simulink model "ex7busLongLine_sim"  (R2014b)
settings: Solver=ode45  SolverMode=SingleTasking  StartTime=0.0  StopTime=5  MaxStep=0.0005  RelTol=1e-07
values from neighbouring files (symbols this model uses):
  bus1_vd = 2^0.5*1e3    (= 1414.21356237)    [ex3busPV.m]    (also in exLongLinePV.m = 141421.356237)
  C2 = 0.1*(len12/NN12+len23/NN23+len25/NN25)*Cx    (= 7.75146666667e-08)    [ex7busLongLine.m]
  C3 = 0.1*(len23/NN23+len34/NN34)*Cx    (= 3.50675e-08)    [ex7busLongLine.m]
  C4 = 0.1*(len14/NN14+len34/NN34+len46/NN46)*Cx    (= 9.28655e-08)    [ex7busLongLine.m]
  C5 = 0.1*(len25/NN25)*Cx    (= 2.39416666667e-08)    [ex7busLongLine.m]
  C6 = 0.1*(len46/NN46+len67/NN67)*Cx    (= 4.85875e-08)    [ex7busLongLine.m]
  C7 = 0.1*(len67/NN67)*Cx    (= 2.66175e-08)    [ex7busLongLine.m]
  CL2 = -CL2    [ex7busLongLine.m]
  CL3 = -CL3    [ex7busLongLine.m]
  CL6 = -CL6    [ex7busLongLine.m]
  CL7 = -CL7    [ex7busLongLine.m]
  DL2 = -DL2    [ex7busLongLine.m]
  DL3 = -DL3    [ex7busLongLine.m]
  DL6 = -DL6    [ex7busLongLine.m]
  DL7 = -DL7    [ex7busLongLine.m]
  droop_Pref = 0.25*Pbase    (= 75000000)    [ex7busLongLine.m]    (also in exDroopA.m = mpc.gen(2:end,PG)*1e6; exDroopB.m = mpc.gen(:,PG)*1e6; exSyncGenPVinv.m = droop_Pref( [1:(synrp-1),(synrp+1):end]  ))
  droop_R = DROOP_R_GAIN_CNST./Prt    [ex7busLongLine.m]    (also in exDroopA.m; exDroopB.m)
  Epv = 22e3    (= 22000)    [ex7busLongLine.m]
  If_dc = 0.2*Prt./Ert    [ex14busSGandPV.m]    (also in ex7busLongLine.m = Prt./(60*Vf_dc); exDroopA.m = Prt./(60*Vf_dc); exDroopB.m = Prt./(60*Vf_dc); exSyncGenPVinv.m)
  Jpv = JPV_CNST*Ppvrt/ws    (= 95.4929658551)    [ex7busLongLine.m]
  Kd = KD_GAIN_CNST*J*ws    [ex14busSGandPV.m]    (also in ex2busStability.m = 24000; ex7busLongLine.m; ex9busSG.m; exDroopA.m)
  Kdpv = KDPV_CNST*Jpv*ws    (= 6000000)    [ex7busLongLine.m]
  L0 = 0.1*Ld    [ex14busSGandPV.m]    (also in ex7busLongLine.m; exDroopA.m; exDroopB.m; exSyncGenPVinv.m)
  Laf = (2^0.5)*Ert./(ws*If_dc)    [ex14busSGandPV.m]    (also in ex7busLongLine.m; exDroopA.m; exDroopB.m; exSyncGenPVinv.m = (2^0.5)*5*Ert.^2./(ws*Prt))
  Lb2 = 2*Ld.*Lff - 3*Laf.^2    [ex14busSGandPV.m]    (also in ex7busLongLine.m; exDroopA.m; exDroopB.m; exSyncGenPVinv.m)
  Ld = 0.6*Lpu    [ex14busSGandPV.m]    (also in ex7busLongLine.m = 0.3*Lpu; exDroopA.m = 0.3*Lpu; exDroopB.m = 0.3*Lpu; exSyncGenPVinv.m)
  Lff = 2*Laf.^2./Ld    [ex14busSGandPV.m]    (also in ex7busLongLine.m; exDroopA.m; exDroopB.m; exSyncGenPVinv.m)
  Lq = Ld    [ex14busSGandPV.m]    (also in ex7busLongLine.m; exDroopA.m; exDroopB.m; exSyncGenPVinv.m)
  Lspv = 0.1*Epv^2/(Ppvrt*ws)    (= 0.00256769974855)    [ex7busLongLine.m]
  PG5 = 0.8*Ppvrt    (= 48000000)    [ex7busLongLine.m]
  poles_2Jws = poles./(2*J*ws)    [ex14busSGandPV.m]    (also in ex2busStability.m = poles./(2*ws*J); ex7busLongLine.m; ex9busSG.m = poles./(2*ws*J); exDroopA.m)
  Ra = 0.05*Ert.^2./Prt    [ex14busSGandPV.m]    (also in ex7busLongLine.m = 0.01*Ert.^2./Prt; exDroopA.m = 0.01*Ert.^2./Prt; exDroopB.m = 0.01*Ert.^2./Prt; exSyncGenPVinv.m)
  rel_step_4 = 0.5    [ex7busLongLine.m]
  rel_step_5 = -0.5    [ex7busLongLine.m]
  Rf = Lff/1.2    [ex14busSGandPV.m]    (also in ex7busLongLine.m = Vf_dc./If_dc; exDroopA.m = Vf_dc./If_dc; exDroopB.m = Vf_dc./If_dc; exSyncGenPVinv.m)
  tratio4 = 22e3 / Vbase    (= 0.136645962733)    [ex7busLongLine.m]
  tratio5 = 22e3 / Vbase    (= 0.136645962733)    [ex7busLongLine.m]
  tss2 = 4.5    [ex7busLongLine.m]
  tss3 = 1e9    (= 1000000000)    [ex7busLongLine.m]
  tss4 = 1e9    (= 1000000000)    [ex7busLongLine.m]
  tss5 = 4    [ex7busLongLine.m]
  tss6 = 1e9    (= 1000000000)    [ex7busLongLine.m]
  tss7 = 1e9    (= 1000000000)    [ex7busLongLine.m]
  Vbase = 161e3    (= 161000)    [ex7busLongLine.m]
  Vf_dc = If_dc.*Rf    [ex14busSGandPV.m]    (also in ex7busLongLine.m = 500 * ones(size(Ert)); exDroopA.m = 500 * ones(size(Ert)); exDroopB.m = 500 * ones(size(Ert)); exSyncGenPVinv.m)
  vinf_0 = 0    [ex14busSGandPV.m]    (also in ex7busLongLine.m; exDroopA.m; exSyncGenPVinv.m)
  vinf_d = (2^0.5)*mpcA.bus(1,VM)*baseV    [ex14busSGandPV.m]    (also in ex7busLongLine.m = 250457.221896; exDroopA.m = (2^0.5)*mpc.bus(1,VM)*baseV(1); exSyncGenPVinv.m = (2^0.5)*mpc.bus(1,VM)*baseV(1))
  vinf_q = 0    [ex14busSGandPV.m]    (also in ex7busLongLine.m; exDroopA.m; exSyncGenPVinv.m)
  ws = 2*pi*50    (= 314.159265359)    [ex14busSGandPV.m]    (also in ex2busStability.m; ex3busPV.m; ex7busLongLine.m; ex9busSG.m)
undefined symbols (not defined in the file or in its folder): AL2, AL3, AL6, AL7, At12, At14, At23, At25, At34, At46, At67, BL2, BL3, BL6, BL7, Bt12, Bt14, Bt23, Bt25, Bt34, Bt46, Bt67, Ct12, Ct14, Ct23, Ct25, Ct34, Ct46, Ct67, Dt12, Dt14, Dt23, Dt25, Dt34, Dt46, Dt67, full
(part 1 of 2)
settings Model: Creator=COPEC  LastModifiedBy=Juri
settings OptimizationCC: BlockReduction=off  BooleanDataType=off
settings DebuggingCC: SaveWithParameterizedLinksMsg=none  UnderspecifiedInitializationDetection=Classic  MergeDetectMultiDrivingBlocksExec=none  SignalResolutionControl=TryResolveAllWithWarning  SolverPrmCheckMsg=none  FrameProcessingCompatibilityMsg=error
settings HardwareCC: TargetUnknown=on

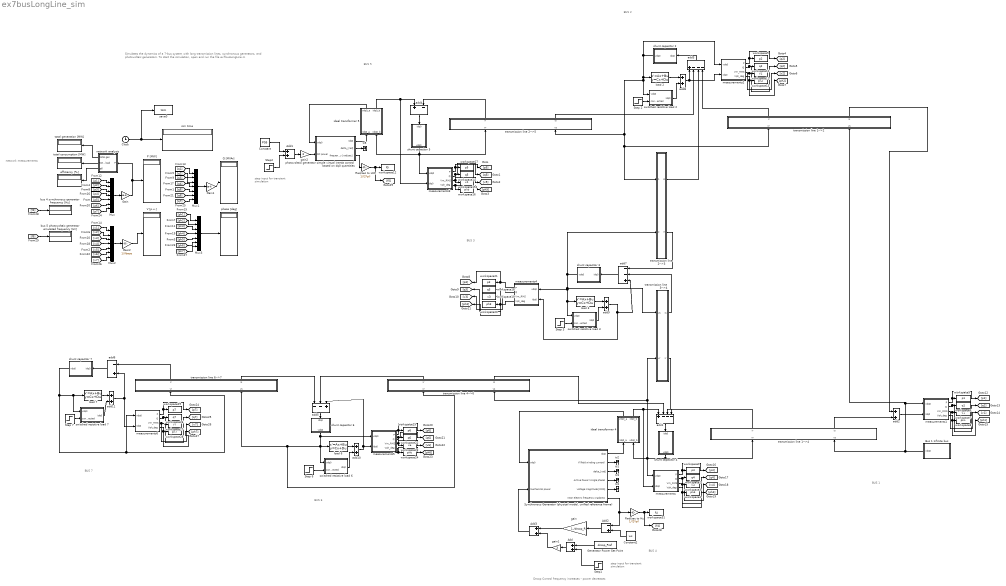
== system ex7busLongLine_sim ==
  note: Simulates the dynamics of a 7-bus system with long transmission lines, synchronous generators, and photovoltaic generators.
      |
      | To start the simulation, open and run the file
      | ex7busLongLine.m
  note: BUS 1
  note: BUS 4
  note: BUS 2
  note: BUS 3
  note: BUS 5
  note: BUS 6
  note: BUS 7
  note: network
      | measurements
  note: Droop Control
      | frequency increases - power decreases
  note: step input
      | for transient simulation
  note: step input
      | for transient simulation
  Add : Sum
  Add1 : Sum
  Add2 : Sum  Inputs=-+
  Add3 : Sum
  Bus 1 Infinite bus : Subsystem
  Clock : Clock
  Constant : Constant  Value=PG5
  Constant2 : Constant  Value=ws
  Gain : Gain  Gain=1e-6
  Gain1 : Gain  Gain=1e-6
  Gain2 : Gain  Gain=1/Vbase
  Generator Power Set Point : Constant  Value=droop_Pref
  Mux{,1..3} (4 alike) : Mux  Inputs=7
  P [MW] : Display
  Q [MVAr] : Display
  Rad/sec to Hz : Gain  Gain=1/(2*pi)
  Rad/sec to Hz1 : Gain  Gain=1/(2*pi)
  Step 2 : Step  Time=tss2  SampleTime=0
  Step 3 : Step  Time=tss3  SampleTime=0
  Step 6 : Step  Time=tss6  SampleTime=0
  Step 7 : Step  Time=tss7  SampleTime=0
  Step1 : Step  Time=tss4  After=rel_step_4*droop_Pref  SampleTime=0
  Step2 : Step  Time=tss5  After=rel_step_5*PG5  SampleTime=0
  "Synchronous Generator (physical model, unified reference frame)" : Subsystem
  V [p.u.] : Display
  add1 : Sum  Inputs=+---
  add{2,8..11} (5 alike) : Sum
  add3 : Sum  Inputs=+---
  add4 : Sum  Inputs=+-
  add5 : Sum  Inputs=--+
  add6 : Sum  Inputs=-+
  add7 : Sum  Inputs=--+
  bus 4 synchronous generator frequency [Hz] : Display
  bus 5 photovoltaic generator emulated frequency [Hz] : Display
  efficiency [%] : Display
  gain : Gain  Gain=1./droop_R
  gain1 : Gain  Gain=3
  gain2 : Gain  Gain=3
  ideal transformer 5 : Subsystem
  ideal transformer 4 : Subsystem
  load 2 : StateSpace  A=full(AL2)  B=full(BL2)  C=full(CL2)  D=full(DL2)  X0=0
  load 3 : StateSpace  A=full(AL3)  B=full(BL3)  C=full(CL3)  D=full(DL3)  X0=0
  load 6 : StateSpace  A=full(AL6)  B=full(BL6)  C=full(CL6)  D=full(DL6)  X0=0
  load 7 : StateSpace  A=full(AL7)  B=full(BL7)  C=full(CL7)  D=full(DL7)  X0=0
  measurements : Subsystem
  measurements1 : Subsystem
  measurements2 : Subsystem
  measurements3 : Subsystem
  measurements4 : Subsystem
  measurements5 : Subsystem
  measurements6 : Subsystem
  network analysis : Subsystem
  phase [deg] : Display
  "photovoltaic generator simple virtual inertia control based on dq0 quantities " : Subsystem
  save0 : ToWorkspace  VariableName=tsim  SampleTime=-1
  shunt capacitor 5 : Subsystem
  shunt capacitor 6 : Subsystem
  shunt capacitor 2 : Subsystem
  shunt capacitor 3 : Subsystem
  shunt capacitor 4 : Subsystem
  shunt capacitor 7 : Subsystem
  sim time : Display
  switched resistive load 2 : Subsystem
  switched resistive load 3 : Subsystem
  switched resistive load 6 : Subsystem
  switched resistive load 7 : Subsystem
  total consumption [MW] : Display
  total generation [MW] : Display
  tr{1..5} (5 alike) : Terminator
  transmission line 1-->2 : Subsystem
  transmission line 1-->4 : Subsystem
  transmission line 2-->3 : Subsystem
  transmission line 2-->5 : Subsystem
  transmission line 3-->4 : Subsystem
  transmission line 4-->6 : Subsystem
  transmission line 6-->7 : Subsystem
  workspace1 : ToWorkspace  VariableName=p4  SampleTime=-1
  workspace10 : ToWorkspace  VariableName=q2  SampleTime=-1
  workspace11 : ToWorkspace  VariableName=v2  SampleTime=-1
  workspace12 : ToWorkspace  VariableName=f5  SampleTime=-1
  workspace13 : ToWorkspace  VariableName=ph2  SampleTime=-1
  workspace14 : ToWorkspace  VariableName=q5  SampleTime=-1
  workspace15 : ToWorkspace  VariableName=v5  SampleTime=-1
  workspace16 : ToWorkspace  VariableName=ph5  SampleTime=-1
  workspace17 : ToWorkspace  VariableName=p5  SampleTime=-1
  workspace18 : ToWorkspace  VariableName=q3  SampleTime=-1
  workspace19 : ToWorkspace  VariableName=v3  SampleTime=-1
  workspace2 : ToWorkspace  VariableName=q4  SampleTime=-1
  workspace20 : ToWorkspace  VariableName=ph3  SampleTime=-1
  workspace21 : ToWorkspace  VariableName=p3  SampleTime=-1
  workspace22 : ToWorkspace  VariableName=q6  SampleTime=-1
  workspace23 : ToWorkspace  VariableName=v6  SampleTime=-1
  workspace24 : ToWorkspace  VariableName=ph6  SampleTime=-1
  workspace25 : ToWorkspace  VariableName=p6  SampleTime=-1
  workspace26 : ToWorkspace  VariableName=q7  SampleTime=-1
  workspace27 : ToWorkspace  VariableName=v7  SampleTime=-1
  workspace28 : ToWorkspace  VariableName=ph7  SampleTime=-1
  workspace29 : ToWorkspace  VariableName=p7  SampleTime=-1
  workspace3 : ToWorkspace  VariableName=v4  SampleTime=-1
  workspace31 : ToWorkspace  VariableName=f4  SampleTime=-1
  workspace4 : ToWorkspace  VariableName=ph4  SampleTime=-1
  workspace5 : ToWorkspace  VariableName=p1  SampleTime=-1
  workspace6 : ToWorkspace  VariableName=q1  SampleTime=-1
  workspace7 : ToWorkspace  VariableName=v1  SampleTime=-1
  workspace8 : ToWorkspace  VariableName=ph1  SampleTime=-1
  workspace9 : ToWorkspace  VariableName=p2  SampleTime=-1
  wires:
  Clock/1 -> save0/1, sim time/1
  "Synchronous Generator (physical model, unified reference frame)"/1(idq0) -> ideal transformer 4/1(idq0_a)
  ideal transformer 4/1(vdq0_a) -> "Synchronous Generator (physical model, unified reference frame)"/1(vdq0)
  shunt capacitor 4/1(vdq0) -> transmission line 1-->4/1(vr), transmission line 4-->6/2(vs), transmission line 3-->4/2(vr), measurements/1(vdq0), ideal transformer 4/2(vdq0_b)
  ideal transformer 4/2(idq0_b) -> measurements/2(idq0), add1/1
  add1/1 -> shunt capacitor 4/1(idq0)
  measurements/1(P) -> [p4], workspace1/1
  measurements/2(Q) -> workspace2/1, [q4]
  measurements/3(Vm_RMS) -> [v4], workspace3/1
  measurements/4(Vph_deg) -> [ph4], workspace4/1
  measurements1/1(P) -> [p1], workspace5/1
  measurements1/2(Q) -> [q1], workspace6/1
  measurements1/3(Vm_RMS) -> [v1], workspace7/1
  measurements1/4(Vph_deg) -> [ph1], workspace8/1
  transmission line 1-->4/2(is) -> add2/2
  Bus 1 Infinite bus/1(vdq0) -> transmission line 1-->4/2(vs), transmission line 1-->2/2(vs), measurements1/1(vdq0)
  transmission line 1-->4/1(ir) -> add1/4
  add2/1 -> measurements1/2(idq0)
  transmission line 3-->4/2(ir) -> add1/3
  transmission line 4-->6/2(is) -> add1/2
  transmission line 1-->2/2(is) -> add2/1
  measurements2/1(P) -> [p2], workspace9/1
  measurements2/2(Q) -> [q2], workspace10/1
  measurements2/3(Vm_RMS) -> [v2], workspace11/1
  measurements2/4(Vph_deg) -> [ph2], workspace13/1
  measurements3/1(P) -> [p5], workspace17/1
  measurements3/2(Q) -> [q5], workspace14/1
  measurements3/3(Vm_RMS) -> workspace15/1, [v5]
  measurements3/4(Vph_deg) -> [ph5], workspace16/1
  measurements4/1(P) -> [p3], workspace21/1
  measurements4/2(Q) -> [q3], workspace18/1
  measurements4/3(Vm_RMS) -> [v3], workspace19/1
  measurements4/4(Vph_deg) -> [ph3], workspace20/1
  measurements5/1(P) -> [p6], workspace25/1
  measurements5/2(Q) -> [q6], workspace22/1
  measurements5/3(Vm_RMS) -> workspace23/1, [v6]
  measurements5/4(Vph_deg) -> [ph6], workspace24/1
  measurements6/1(P) -> [p7], workspace29/1
  measurements6/2(Q) -> [q7], workspace26/1
  measurements6/3(Vm_RMS) -> workspace27/1, [v7]
  measurements6/4(Vph_deg) -> [ph7], workspace28/1
  add4/1 -> shunt capacitor 5/1(idq0)
  shunt capacitor 5/1(vdq0) -> measurements3/1(vdq0), transmission line 2-->5/1(vr), ideal transformer 5/2(vdq0_b)
  ideal transformer 5/2(idq0_b) -> measurements3/2(idq0), add4/1
  transmission line 2-->5/1(ir) -> add4/2
  add3/1 -> shunt capacitor 2/1(idq0)
  shunt capacitor 2/1(vdq0) -> switched resistive load 2/1(vdq0), transmission line 1-->2/1(vr), transmission line 2-->3/1(vs), transmission line 2-->5/2(vs), load 2/1, measurements2/1(vdq0)
  add8/1 -> measurements2/2(idq0), add3/1
  transmission line 2-->5/2(is) -> add3/2
  transmission line 1-->2/1(ir) -> add3/4
  transmission line 2-->3/1(is) -> add3/3
  add9/1 -> measurements4/2(idq0), add7/3
  add7/1 -> shunt capacitor 3/1(idq0)
  transmission line 3-->4/1(is) -> add7/2
  transmission line 2-->3/2(ir) -> add7/1
  shunt capacitor 3/1(vdq0) -> switched resistive load 3/1(vdq0), load 3/1, measurements4/1(vdq0), transmission line 3-->4/1(vs), transmission line 2-->3/2(vr)
  add5/1 -> shunt capacitor 6/1(idq0)
  shunt capacitor 6/1(vdq0) -> switched resistive load 6/1(vdq0), load 6/1, transmission line 6-->7/2(vs), transmission line 4-->6/1(vr), measurements5/1(vdq0)
  add10/1 -> measurements5/2(idq0), add5/3
  transmission line 4-->6/1(ir) -> add5/2
  transmission line 6-->7/2(is) -> add5/1
  add6/1 -> shunt capacitor 7/1(idq0)
  transmission line 6-->7/1(ir) -> add6/1
  add11/1 -> measurements6/2(idq0), add6/2
  shunt capacitor 7/1(vdq0) -> load 7/1, switched resistive load 7/1(vdq0), measurements6/1(vdq0), transmission line 6-->7/1(vr)
  [p1] -> Mux/1
  [p2] -> Mux/2
  [p3] -> Mux/3
  [p4] -> Mux/4
  [p5] -> Mux/5
  [p6] -> Mux/6
  [p7] -> Mux/7
  [q1] -> Mux1/1
  [q2] -> Mux1/2
  [q3] -> Mux1/3
  [q4] -> Mux1/4
  [q5] -> Mux1/5
  [q6] -> Mux1/6
  [q7] -> Mux1/7
  [v1] -> Mux2/1
  [v2] -> Mux2/2
  [v3] -> Mux2/3
  [v4] -> Mux2/4
  [v5] -> Mux2/5
  [v6] -> Mux2/6
  [v7] -> Mux2/7
  [ph1] -> Mux3/1
  [ph2] -> Mux3/2
  [ph3] -> Mux3/3
  [ph4] -> Mux3/4
  [ph5] -> Mux3/5
  [ph6] -> Mux3/6
  [ph7] -> Mux3/7
  Mux/1 -> Gain/1
  Mux1/1 -> Gain1/1
  Mux2/1 -> Gain2/1
  Gain/1 -> network analysis/1(P), P [MW]/1
  Gain1/1 -> Q [MVAr]/1
  Gain2/1 -> V [p.u.]/1
  Mux3/1 -> phase [deg]/1
  "photovoltaic generator simple virtual inertia control based on dq0 quantities "/1(idq0) -> ideal transformer 5/1(idq0_a)
  network analysis/3(eff) -> efficiency [%]/1
  network analysis/2(total load) -> total consumption [MW]/1
  network analysis/1(total gen) -> total generation [MW]/1
  "Synchronous Generator (physical model, unified reference frame)"/2(if (field winding current)) -> tr2/1
  "Synchronous Generator (physical model, unified reference frame)"/3(delta_[rad]) -> tr1/1
  "Synchronous Generator (physical model, unified reference frame)"/6(rotor electric frequency [rad/sec]) -> Rad/sec to Hz/1, Add2/1
  Rad/sec to Hz/1 -> [f4], workspace31/1
  "Synchronous Generator (physical model, unified reference frame)"/4(Active Power (single phase)) -> tr3/1
  "Synchronous Generator (physical model, unified reference frame)"/5(voltage magnitude [RMS]) -> tr4/1
  Constant2/1 -> Add2/2
  Add2/1 -> gain/1
  gain1/1 -> Add3/2
  gain/1 -> Add3/1
  Add3/1 -> "Synchronous Generator (physical model, unified reference frame)"/2(mechanical power)
  [f4] -> bus 4 synchronous generator frequency [Hz]/1
  ideal transformer 5/1(vdq0_a) -> "photovoltaic generator simple virtual inertia control based on dq0 quantities "/1(vdq0)
  gain2/1 -> "photovoltaic generator simple virtual inertia control based on dq0 quantities "/2(DC power)
  Constant/1 -> Add1/1
  Rad/sec to Hz1/1 -> [f5], workspace12/1
  "photovoltaic generator simple virtual inertia control based on dq0 quantities "/2(delta_[rad]) -> tr5/1
  [f5] -> bus 5 photovoltaic generator emulated frequency [Hz]/1
  "photovoltaic generator simple virtual inertia control based on dq0 quantities "/3(frequency [rad/sec]) -> Rad/sec to Hz1/1
  switched resistive load 2/1(idq0) -> add8/2
  load 2/1 -> add8/1
  Step 2/1 -> switched resistive load 2/2(connected)
  load 3/1 -> add9/1
  switched resistive load 3/1(idq0) -> add9/2
  Step 3/1 -> switched resistive load 3/2(connected)
  load 6/1 -> add10/1
  switched resistive load 6/1(idq0) -> add10/2
  Step 6/1 -> switched resistive load 6/2(connected)
  load 7/1 -> add11/1
  Step 7/1 -> switched resistive load 7/2(connected)
  switched resistive load 7/1(idq0) -> add11/2
  Add/1 -> gain1/1
  Generator Power Set Point/1 -> Add/1
  Step1/1 -> Add/2
  Add1/1 -> gain2/1
  Step2/1 -> Add1/2

== system ex7busLongLine_sim/Bus 1 Infinite bus ==
  Constant : Constant  Value=vinf_d
  Constant1 : Constant  Value=vinf_q
  Constant2 : Constant  Value=vinf_0
  Mux1 : Mux  Inputs=3
  vdq0 : Outport
  wires:
  Mux1/1 -> vdq0/1
  Constant/1 -> Mux1/1
  Constant1/1 -> Mux1/2
  Constant2/1 -> Mux1/3

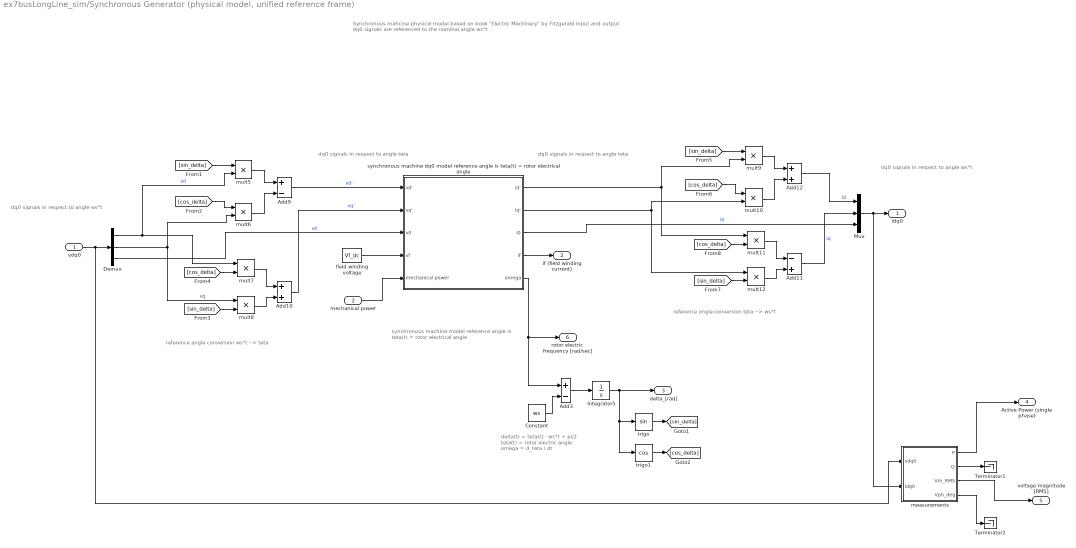
== system ex7busLongLine_sim/Synchronous Generator (physical model, unified reference frame) ==
  note: Synchronous mahcine physical model
      | based on book "Electric Machinery" by Fitzgerald
      |
      | input and output dq0 signals are referenced
      | to the nominal angle ws*t
  note: reference angle conversion ws*t --> teta
  note: synchronous machine model
      | reference angle is
      | teta(t) = rotor electrical angle
  note: reference angle conversion teta --> ws*t
  note: dq0 signals in respect to angle ws*t
  note: dq0 signals in respect to angle ws*t
  note: dq0 signals in respect to angle teta
  note: dq0 signals in respect to angle teta
  note: delta(t) = teta(t) - ws*t + pi/2
      | teta(t) = rotor electric angle
      | omega = d_teta / dt
  vdq0 : Inport
  mechanical power : Inport  Port=2
  Add10 : Sum
  Add11 : Sum  Inputs=-+
  Add12 : Sum
  Add3 : Sum  Inputs=+-
  Add9 : Sum  Inputs=+-
  Constant : Constant  Value=ws
  Demux : Demux  Outputs=3
  Integrator5 : Integrator
  Mux : Mux  Inputs=3
  Terminator1 : Terminator
  Terminator2 : Terminator
  field winding voltage : Constant  Value=Vf_dc
  measurements : Subsystem
  mult{5..12} (8 alike) : Product  Inputs=**
  synchronous machine dq0 model reference angle is teta(t) = rotor electrical angle : Subsystem
  trigo : Trigonometry
  trigo1 : Trigonometry  Operator=cos
  idq0 : Outport
  if (field winding current) : Outport  Port=2
  delta_[rad] : Outport  Port=3
  Active Power (single phase) : Outport  Port=4
  voltage magnitude [RMS] : Outport  Port=5
  rotor electric frequency [rad/sec] : Outport  Port=6
  wires:
  vdq0/1 -> measurements/1(vdq0), Demux/1
  Demux/1 -> mult5/2, mult7/1  "vd"
  Demux/2 -> mult6/2, mult8/1  "vq"
  mult5/1 -> Add9/1
  mult6/1 -> Add9/2
  [sin_delta] -> mult5/1
  [cos_delta] -> mult6/1
  mult7/1 -> Add10/1
  mult8/1 -> Add10/2
  [cos_delta] -> mult7/2
  [sin_delta] -> mult8/2
  mult9/1 -> Add12/1
  mult10/1 -> Add12/2
  [sin_delta] -> mult9/1
  [cos_delta] -> mult10/1
  mult11/1 -> Add11/1
  mult12/1 -> Add11/2
  [cos_delta] -> mult11/2
  [sin_delta] -> mult12/2
  Mux/1 -> measurements/2(idq0), idq0/1
  Add11/1 -> Mux/2  "iq"
  Add12/1 -> Mux/1  "id"
  synchronous machine dq0 model reference angle is teta(t) = rotor electrical angle/1(id') -> mult11/1, mult9/2
  synchronous machine dq0 model reference angle is teta(t) = rotor electrical angle/2(iq') -> mult12/1, mult10/2
  Add9/1 -> synchronous machine dq0 model reference angle is teta(t) = rotor electrical angle/1(vd')  "vd'"
  mechanical power/1 -> synchronous machine dq0 model reference angle is teta(t) = rotor electrical angle/5(mechanical power)
  Demux/3 -> synchronous machine dq0 model reference angle is teta(t) = rotor electrical angle/3(v0)  "v0"
  Add10/1 -> synchronous machine dq0 model reference angle is teta(t) = rotor electrical angle/2(vq')  "vq'"
  field winding voltage/1 -> synchronous machine dq0 model reference angle is teta(t) = rotor electrical angle/4(vf)
  synchronous machine dq0 model reference angle is teta(t) = rotor electrical angle/3(i0) -> Mux/3  "i0"
  synchronous machine dq0 model reference angle is teta(t) = rotor electrical angle/4(if) -> if (field winding current)/1
  trigo/1 -> [sin_delta]
  trigo1/1 -> [cos_delta]
  Add3/1 -> Integrator5/1
  Constant/1 -> Add3/2
  synchronous machine dq0 model reference angle is teta(t) = rotor electrical angle/5(omega) -> Add3/1, rotor electric frequency [rad/sec]/1
  Integrator5/1 -> delta_[rad]/1, trigo1/1, trigo/1
  measurements/1(P) -> Active Power (single phase)/1
  measurements/2(Q) -> Terminator1/1
  measurements/3(Vm_RMS) -> voltage magnitude [RMS]/1
  measurements/4(Vph_deg) -> Terminator2/1

== system ex7busLongLine_sim/ideal transformer 5 ==
  idq0_a : Inport
  vdq0_b : Inport  Port=2
  gain1 : Gain  Gain=tratio5
  gain2 : Gain  Gain=tratio5
  vdq0_a : Outport
  idq0_b : Outport  Port=2
  wires:
  vdq0_b/1 -> gain1/1
  gain1/1 -> vdq0_a/1
  idq0_a/1 -> gain2/1
  gain2/1 -> idq0_b/1

== system ex7busLongLine_sim/ideal transformer 4 ==
  idq0_a : Inport
  vdq0_b : Inport  Port=2
  gain1 : Gain  Gain=tratio4
  gain2 : Gain  Gain=tratio4
  vdq0_a : Outport
  idq0_b : Outport  Port=2
  wires:
  vdq0_b/1 -> gain1/1
  gain1/1 -> vdq0_a/1
  idq0_a/1 -> gain2/1
  gain2/1 -> idq0_b/1

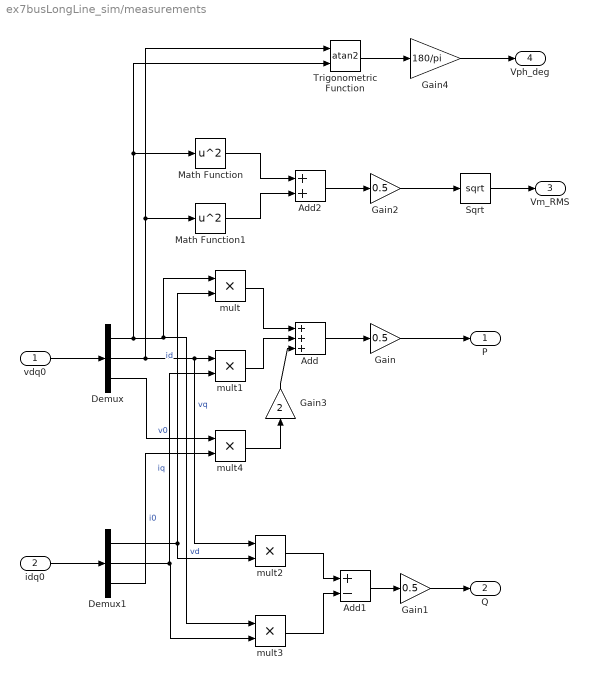
== system ex7busLongLine_sim/measurements ==
  vdq0 : Inport
  idq0 : Inport  Port=2
  Add : Sum  Inputs=+++
  Add1 : Sum  Inputs=+-
  Add2 : Sum
  Demux : Demux  Outputs=3
  Demux1 : Demux  Outputs=3
  Gain : Gain  Gain=0.5
  Gain1 : Gain  Gain=0.5
  Gain2 : Gain  Gain=0.5
  Gain3 : Gain  Gain=2
  Gain4 : Gain  Gain=180/pi
  Math Function : Math  Operator=square  SaturateOnIntegerOverflow=on
  Math Function1 : Math  Operator=square  SaturateOnIntegerOverflow=on
  Sqrt : Sqrt  SaturateOnIntegerOverflow=on
  Trigonometric Function : Trigonometry  Operator=atan2
  mult{,1..4} (5 alike) : Product  Inputs=**
  P : Outport
  Q : Outport  Port=2
  Vm_RMS : Outport  Port=3
  Vph_deg : Outport  Port=4
  wires:
  idq0/1 -> Demux1/1
  vdq0/1 -> Demux/1
  Demux/1 -> Math Function/1, Trigonometric Function/2, mult3/1, mult/1  "vd"
  Demux/2 -> Trigonometric Function/1, Math Function1/1, mult2/1, mult1/1  "vq"
  Demux1/1 -> mult/2, mult2/2  "id"
  Demux1/2 -> mult3/2, mult1/2  "iq"
  Demux/3 -> mult4/1  "v0"
  Demux1/3 -> mult4/2  "i0"
  mult/1 -> Add/1
  mult1/1 -> Add/2
  Add/1 -> Gain/1
  mult2/1 -> Add1/1
  mult3/1 -> Add1/2
  Add1/1 -> Gain1/1
  Sqrt/1 -> Vm_RMS/1
  Math Function/1 -> Add2/1
  Math Function1/1 -> Add2/2
  Add2/1 -> Gain2/1
  Gain2/1 -> Sqrt/1
  Gain/1 -> P/1
  Gain1/1 -> Q/1
  mult4/1 -> Gain3/1
  Gain3/1 -> Add/3
  Trigonometric Function/1 -> Gain4/1
  Gain4/1 -> Vph_deg/1

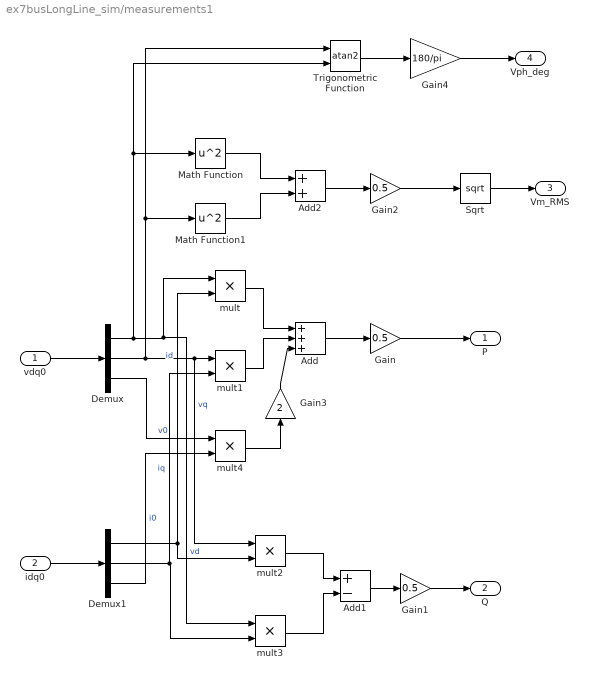
== system ex7busLongLine_sim/measurements1 ==
  vdq0 : Inport
  idq0 : Inport  Port=2
  Add : Sum  Inputs=+++
  Add1 : Sum  Inputs=+-
  Add2 : Sum
  Demux : Demux  Outputs=3
  Demux1 : Demux  Outputs=3
  Gain : Gain  Gain=0.5
  Gain1 : Gain  Gain=0.5
  Gain2 : Gain  Gain=0.5
  Gain3 : Gain  Gain=2
  Gain4 : Gain  Gain=180/pi
  Math Function : Math  Operator=square  SaturateOnIntegerOverflow=on
  Math Function1 : Math  Operator=square  SaturateOnIntegerOverflow=on
  Sqrt : Sqrt  SaturateOnIntegerOverflow=on
  Trigonometric Function : Trigonometry  Operator=atan2
  mult{,1..4} (5 alike) : Product  Inputs=**
  P : Outport
  Q : Outport  Port=2
  Vm_RMS : Outport  Port=3
  Vph_deg : Outport  Port=4
  wires:
  idq0/1 -> Demux1/1
  vdq0/1 -> Demux/1
  Demux/1 -> Math Function/1, Trigonometric Function/2, mult3/1, mult/1  "vd"
  Demux/2 -> Trigonometric Function/1, Math Function1/1, mult2/1, mult1/1  "vq"
  Demux1/1 -> mult/2, mult2/2  "id"
  Demux1/2 -> mult3/2, mult1/2  "iq"
  Demux/3 -> mult4/1  "v0"
  Demux1/3 -> mult4/2  "i0"
  mult/1 -> Add/1
  mult1/1 -> Add/2
  Add/1 -> Gain/1
  mult2/1 -> Add1/1
  mult3/1 -> Add1/2
  Add1/1 -> Gain1/1
  Sqrt/1 -> Vm_RMS/1
  Math Function/1 -> Add2/1
  Math Function1/1 -> Add2/2
  Add2/1 -> Gain2/1
  Gain2/1 -> Sqrt/1
  Gain/1 -> P/1
  Gain1/1 -> Q/1
  mult4/1 -> Gain3/1
  Gain3/1 -> Add/3
  Trigonometric Function/1 -> Gain4/1
  Gain4/1 -> Vph_deg/1

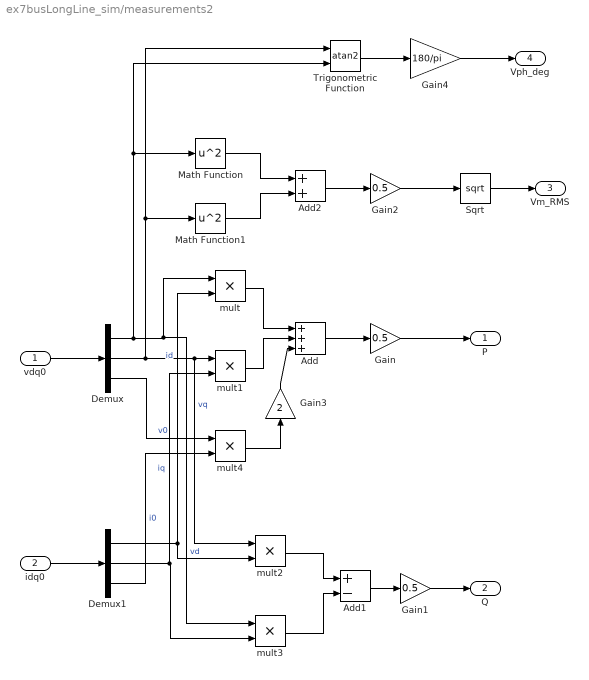
== system ex7busLongLine_sim/measurements2 ==
  vdq0 : Inport
  idq0 : Inport  Port=2
  Add : Sum  Inputs=+++
  Add1 : Sum  Inputs=+-
  Add2 : Sum
  Demux : Demux  Outputs=3
  Demux1 : Demux  Outputs=3
  Gain : Gain  Gain=0.5
  Gain1 : Gain  Gain=0.5
  Gain2 : Gain  Gain=0.5
  Gain3 : Gain  Gain=2
  Gain4 : Gain  Gain=180/pi
  Math Function : Math  Operator=square  SaturateOnIntegerOverflow=on
  Math Function1 : Math  Operator=square  SaturateOnIntegerOverflow=on
  Sqrt : Sqrt  SaturateOnIntegerOverflow=on
  Trigonometric Function : Trigonometry  Operator=atan2
  mult{,1..4} (5 alike) : Product  Inputs=**
  P : Outport
  Q : Outport  Port=2
  Vm_RMS : Outport  Port=3
  Vph_deg : Outport  Port=4
  wires:
  idq0/1 -> Demux1/1
  vdq0/1 -> Demux/1
  Demux/1 -> Math Function/1, Trigonometric Function/2, mult3/1, mult/1  "vd"
  Demux/2 -> Trigonometric Function/1, Math Function1/1, mult2/1, mult1/1  "vq"
  Demux1/1 -> mult/2, mult2/2  "id"
  Demux1/2 -> mult3/2, mult1/2  "iq"
  Demux/3 -> mult4/1  "v0"
  Demux1/3 -> mult4/2  "i0"
  mult/1 -> Add/1
  mult1/1 -> Add/2
  Add/1 -> Gain/1
  mult2/1 -> Add1/1
  mult3/1 -> Add1/2
  Add1/1 -> Gain1/1
  Sqrt/1 -> Vm_RMS/1
  Math Function/1 -> Add2/1
  Math Function1/1 -> Add2/2
  Add2/1 -> Gain2/1
  Gain2/1 -> Sqrt/1
  Gain/1 -> P/1
  Gain1/1 -> Q/1
  mult4/1 -> Gain3/1
  Gain3/1 -> Add/3
  Trigonometric Function/1 -> Gain4/1
  Gain4/1 -> Vph_deg/1

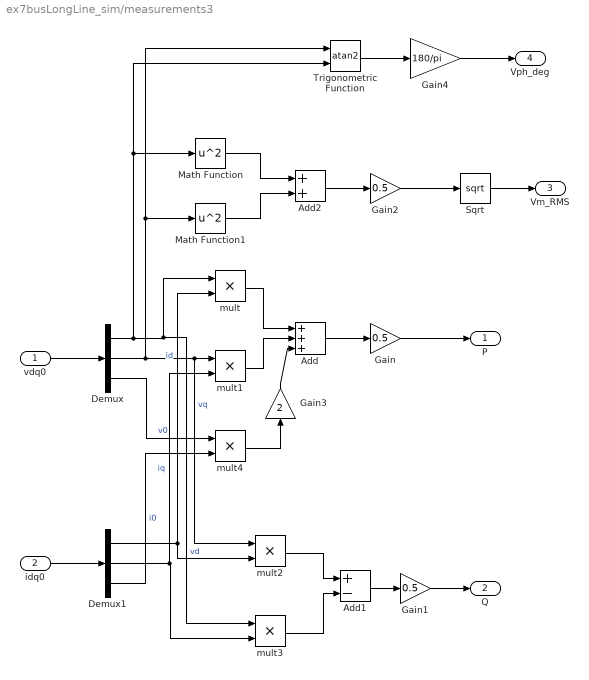
== system ex7busLongLine_sim/measurements3 ==
  vdq0 : Inport
  idq0 : Inport  Port=2
  Add : Sum  Inputs=+++
  Add1 : Sum  Inputs=+-
  Add2 : Sum
  Demux : Demux  Outputs=3
  Demux1 : Demux  Outputs=3
  Gain : Gain  Gain=0.5
  Gain1 : Gain  Gain=0.5
  Gain2 : Gain  Gain=0.5
  Gain3 : Gain  Gain=2
  Gain4 : Gain  Gain=180/pi
  Math Function : Math  Operator=square  SaturateOnIntegerOverflow=on
  Math Function1 : Math  Operator=square  SaturateOnIntegerOverflow=on
  Sqrt : Sqrt  SaturateOnIntegerOverflow=on
  Trigonometric Function : Trigonometry  Operator=atan2
  mult{,1..4} (5 alike) : Product  Inputs=**
  P : Outport
  Q : Outport  Port=2
  Vm_RMS : Outport  Port=3
  Vph_deg : Outport  Port=4
  wires:
  idq0/1 -> Demux1/1
  vdq0/1 -> Demux/1
  Demux/1 -> Math Function/1, Trigonometric Function/2, mult3/1, mult/1  "vd"
  Demux/2 -> Trigonometric Function/1, Math Function1/1, mult2/1, mult1/1  "vq"
  Demux1/1 -> mult/2, mult2/2  "id"
  Demux1/2 -> mult3/2, mult1/2  "iq"
  Demux/3 -> mult4/1  "v0"
  Demux1/3 -> mult4/2  "i0"
  mult/1 -> Add/1
  mult1/1 -> Add/2
  Add/1 -> Gain/1
  mult2/1 -> Add1/1
  mult3/1 -> Add1/2
  Add1/1 -> Gain1/1
  Sqrt/1 -> Vm_RMS/1
  Math Function/1 -> Add2/1
  Math Function1/1 -> Add2/2
  Add2/1 -> Gain2/1
  Gain2/1 -> Sqrt/1
  Gain/1 -> P/1
  Gain1/1 -> Q/1
  mult4/1 -> Gain3/1
  Gain3/1 -> Add/3
  Trigonometric Function/1 -> Gain4/1
  Gain4/1 -> Vph_deg/1

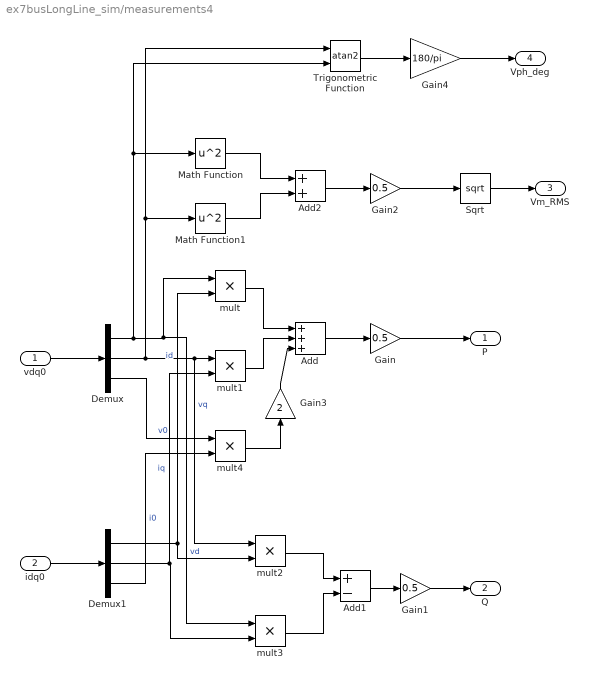
== system ex7busLongLine_sim/measurements4 ==
  vdq0 : Inport
  idq0 : Inport  Port=2
  Add : Sum  Inputs=+++
  Add1 : Sum  Inputs=+-
  Add2 : Sum
  Demux : Demux  Outputs=3
  Demux1 : Demux  Outputs=3
  Gain : Gain  Gain=0.5
  Gain1 : Gain  Gain=0.5
  Gain2 : Gain  Gain=0.5
  Gain3 : Gain  Gain=2
  Gain4 : Gain  Gain=180/pi
  Math Function : Math  Operator=square  SaturateOnIntegerOverflow=on
  Math Function1 : Math  Operator=square  SaturateOnIntegerOverflow=on
  Sqrt : Sqrt  SaturateOnIntegerOverflow=on
  Trigonometric Function : Trigonometry  Operator=atan2
  mult{,1..4} (5 alike) : Product  Inputs=**
  P : Outport
  Q : Outport  Port=2
  Vm_RMS : Outport  Port=3
  Vph_deg : Outport  Port=4
  wires:
  idq0/1 -> Demux1/1
  vdq0/1 -> Demux/1
  Demux/1 -> Math Function/1, Trigonometric Function/2, mult3/1, mult/1  "vd"
  Demux/2 -> Trigonometric Function/1, Math Function1/1, mult2/1, mult1/1  "vq"
  Demux1/1 -> mult/2, mult2/2  "id"
  Demux1/2 -> mult3/2, mult1/2  "iq"
  Demux/3 -> mult4/1  "v0"
  Demux1/3 -> mult4/2  "i0"
  mult/1 -> Add/1
  mult1/1 -> Add/2
  Add/1 -> Gain/1
  mult2/1 -> Add1/1
  mult3/1 -> Add1/2
  Add1/1 -> Gain1/1
  Sqrt/1 -> Vm_RMS/1
  Math Function/1 -> Add2/1
  Math Function1/1 -> Add2/2
  Add2/1 -> Gain2/1
  Gain2/1 -> Sqrt/1
  Gain/1 -> P/1
  Gain1/1 -> Q/1
  mult4/1 -> Gain3/1
  Gain3/1 -> Add/3
  Trigonometric Function/1 -> Gain4/1
  Gain4/1 -> Vph_deg/1

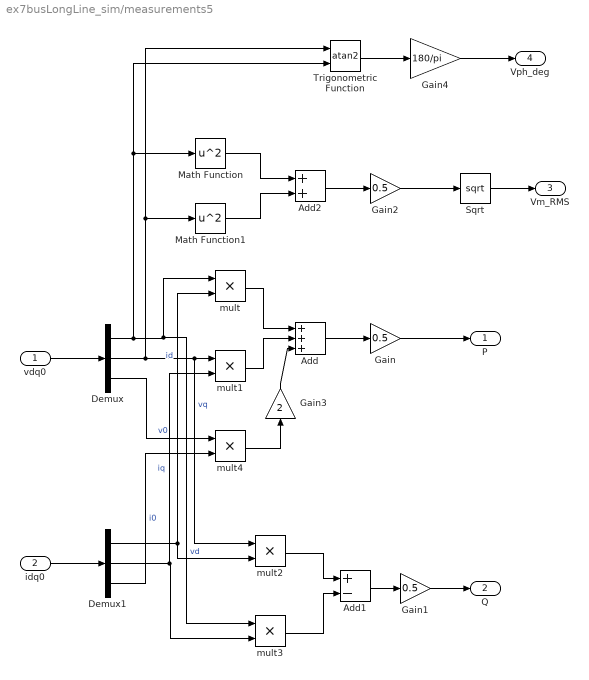
== system ex7busLongLine_sim/measurements5 ==
  vdq0 : Inport
  idq0 : Inport  Port=2
  Add : Sum  Inputs=+++
  Add1 : Sum  Inputs=+-
  Add2 : Sum
  Demux : Demux  Outputs=3
  Demux1 : Demux  Outputs=3
  Gain : Gain  Gain=0.5
  Gain1 : Gain  Gain=0.5
  Gain2 : Gain  Gain=0.5
  Gain3 : Gain  Gain=2
  Gain4 : Gain  Gain=180/pi
  Math Function : Math  Operator=square  SaturateOnIntegerOverflow=on
  Math Function1 : Math  Operator=square  SaturateOnIntegerOverflow=on
  Sqrt : Sqrt  SaturateOnIntegerOverflow=on
  Trigonometric Function : Trigonometry  Operator=atan2
  mult{,1..4} (5 alike) : Product  Inputs=**
  P : Outport
  Q : Outport  Port=2
  Vm_RMS : Outport  Port=3
  Vph_deg : Outport  Port=4
  wires:
  idq0/1 -> Demux1/1
  vdq0/1 -> Demux/1
  Demux/1 -> Math Function/1, Trigonometric Function/2, mult3/1, mult/1  "vd"
  Demux/2 -> Trigonometric Function/1, Math Function1/1, mult2/1, mult1/1  "vq"
  Demux1/1 -> mult/2, mult2/2  "id"
  Demux1/2 -> mult3/2, mult1/2  "iq"
  Demux/3 -> mult4/1  "v0"
  Demux1/3 -> mult4/2  "i0"
  mult/1 -> Add/1
  mult1/1 -> Add/2
  Add/1 -> Gain/1
  mult2/1 -> Add1/1
  mult3/1 -> Add1/2
  Add1/1 -> Gain1/1
  Sqrt/1 -> Vm_RMS/1
  Math Function/1 -> Add2/1
  Math Function1/1 -> Add2/2
  Add2/1 -> Gain2/1
  Gain2/1 -> Sqrt/1
  Gain/1 -> P/1
  Gain1/1 -> Q/1
  mult4/1 -> Gain3/1
  Gain3/1 -> Add/3
  Trigonometric Function/1 -> Gain4/1
  Gain4/1 -> Vph_deg/1

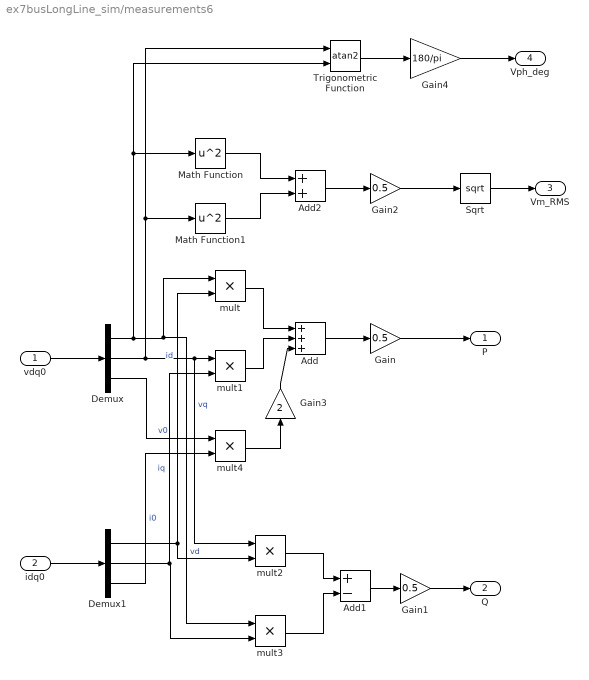
== system ex7busLongLine_sim/measurements6 ==
  vdq0 : Inport
  idq0 : Inport  Port=2
  Add : Sum  Inputs=+++
  Add1 : Sum  Inputs=+-
  Add2 : Sum
  Demux : Demux  Outputs=3
  Demux1 : Demux  Outputs=3
  Gain : Gain  Gain=0.5
  Gain1 : Gain  Gain=0.5
  Gain2 : Gain  Gain=0.5
  Gain3 : Gain  Gain=2
  Gain4 : Gain  Gain=180/pi
  Math Function : Math  Operator=square  SaturateOnIntegerOverflow=on
  Math Function1 : Math  Operator=square  SaturateOnIntegerOverflow=on
  Sqrt : Sqrt  SaturateOnIntegerOverflow=on
  Trigonometric Function : Trigonometry  Operator=atan2
  mult{,1..4} (5 alike) : Product  Inputs=**
  P : Outport
  Q : Outport  Port=2
  Vm_RMS : Outport  Port=3
  Vph_deg : Outport  Port=4
  wires:
  idq0/1 -> Demux1/1
  vdq0/1 -> Demux/1
  Demux/1 -> Math Function/1, Trigonometric Function/2, mult3/1, mult/1  "vd"
  Demux/2 -> Trigonometric Function/1, Math Function1/1, mult2/1, mult1/1  "vq"
  Demux1/1 -> mult/2, mult2/2  "id"
  Demux1/2 -> mult3/2, mult1/2  "iq"
  Demux/3 -> mult4/1  "v0"
  Demux1/3 -> mult4/2  "i0"
  mult/1 -> Add/1
  mult1/1 -> Add/2
  Add/1 -> Gain/1
  mult2/1 -> Add1/1
  mult3/1 -> Add1/2
  Add1/1 -> Gain1/1
  Sqrt/1 -> Vm_RMS/1
  Math Function/1 -> Add2/1
  Math Function1/1 -> Add2/2
  Add2/1 -> Gain2/1
  Gain2/1 -> Sqrt/1
  Gain/1 -> P/1
  Gain1/1 -> Q/1
  mult4/1 -> Gain3/1
  Gain3/1 -> Add/3
  Trigonometric Function/1 -> Gain4/1
  Gain4/1 -> Vph_deg/1

== system ex7busLongLine_sim/network analysis ==
  P : Inport
  Divide : Product  Inputs=/*
  Gain1 : Gain  Gain=100
  Gain4 : Gain  Gain=-1
  Saturation : Saturate  UpperLimit=inf  LowerLimit=1e-9  ZeroCross=off
  Saturation1 : Saturate  UpperLimit=inf  LowerLimit=0  ZeroCross=off
  Sum : Sum  Inputs=+
  Sum1 : Sum  Inputs=+
  total gen : Outport
  total load : Outport  Port=2
  eff : Outport  Port=3
  wires:
  Sum/1 -> total gen/1, Divide/1
  Gain4/1 -> Saturation1/1
  Saturation/1 -> Sum/1
  Saturation1/1 -> Sum1/1
  Sum1/1 -> total load/1, Divide/2
  P/1 -> Gain4/1, Saturation/1
  Gain1/1 -> eff/1
  Divide/1 -> Gain1/1

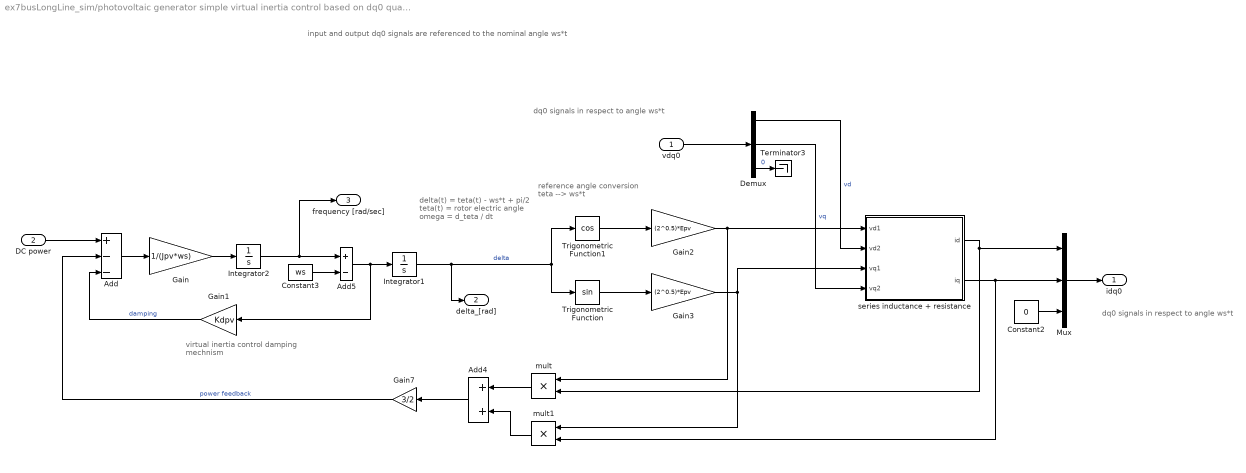
== system ex7busLongLine_sim/photovoltaic generator simple virtual inertia control based on dq0 quantities  ==
  note: reference angle conversion
      | teta --> ws*t
  note: delta(t) = teta(t) - ws*t + pi/2
      | teta(t) = rotor electric angle
      | omega = d_teta / dt
  note: dq0 signals in respect to angle ws*t
  note: dq0 signals in respect to angle ws*t
  note: input and output dq0 signals are referenced
      | to the nominal angle ws*t
  note: virtual inertia control
      | damping mechnism
  vdq0 : Inport
  DC power : Inport  Port=2
  Add : Sum  Inputs=+--
  Add4 : Sum
  Add5 : Sum  Inputs=+-
  Constant2 : Constant  Value=0
  Constant3 : Constant  Value=ws
  Demux : Demux  Outputs=3
  Gain : Gain  Gain=1/(Jpv*ws)
  Gain1 : Gain  Gain=Kdpv
  Gain2 : Gain  Gain=(2^0.5)*Epv
  Gain3 : Gain  Gain=(2^0.5)*Epv
  Gain7 : Gain  Gain=3/2
  Integrator1 : Integrator
  Integrator2 : Integrator  InitialCondition=ws
  Mux : Mux  Inputs=3
  Terminator3 : Terminator
  Trigonometric Function : Trigonometry
  Trigonometric Function1 : Trigonometry  Operator=cos
  mult : Product  Inputs=**
  mult1 : Product  Inputs=**
  series inductance + resistance : Subsystem
  idq0 : Outport
  delta_[rad] : Outport  Port=2
  frequency [rad/sec] : Outport  Port=3
  wires:
  DC power/1 -> Add/1
  Add/1 -> Gain/1
  Gain/1 -> Integrator2/1
  Integrator1/1 -> delta_[rad]/1, Trigonometric Function1/1, Trigonometric Function/1  "delta"
  mult/1 -> Add4/1
  mult1/1 -> Add4/2
  Add4/1 -> Gain7/1
  Gain7/1 -> Add/2  "power feedback"
  Constant2/1 -> Mux/3
  Gain2/1 -> mult/1, series inductance + resistance/1(vd1)
  Gain3/1 -> mult1/1, series inductance + resistance/3(vq1)
  vdq0/1 -> Demux/1
  Demux/1 -> series inductance + resistance/2(vd2)  "vd"
  Demux/2 -> series inductance + resistance/4(vq2)  "vq"
  Demux/3 -> Terminator3/1  "0"
  Mux/1 -> idq0/1
  series inductance + resistance/1(id) -> mult/2, Mux/1
  series inductance + resistance/2(iq) -> mult1/2, Mux/2
  Integrator2/1 -> Add5/1, frequency [rad/sec]/1
  Constant3/1 -> Add5/2
  Trigonometric Function1/1 -> Gain2/1
  Trigonometric Function/1 -> Gain3/1
  Gain1/1 -> Add/3  "damping"
  Add5/1 -> Gain1/1, Integrator1/1

== system ex7busLongLine_sim/shunt capacitor 5 ==
  note: dynamic model of balanced three-phase shunt capacitor unit, based on dq0 signals.
      | idq0 is the current flowing into the capacitor.
      | vdq0 is the capacitor voltage .
      | C is the capacitance (usually in F).
      | initial voltage - initial voltage on the capacitor (dq0 components).
  idq0 : Inport
  1 / capacitance value 0 : Gain  Gain=1/C5
  1 / capacitance value d : Gain  Gain=1/C5
  1 / capacitance value q : Gain  Gain=1/C5
  Add : Sum
  Add1 : Sum  Inputs=-+
  Constant : Constant  Value=(2^0.5)*Vbase
  Constant1 : Constant  Value=0
  Constant2 : Constant  Value=0
  Demux : Demux  Outputs=3
  Gain1 : Gain  Gain=ws
  Gain2 : Gain  Gain=ws
  Integrator : Integrator  InitialConditionSource=external  InitialCondition=bus1_vd
  Integrator1 : Integrator  InitialConditionSource=external  InitialCondition=bus1_vd
  Integrator3 : Integrator  InitialConditionSource=external  InitialCondition=bus1_vd
  Mux : Mux  Inputs=3
  vdq0 : Outport
  wires:
  Integrator1/1 -> Mux/3  "v0"
  Mux/1 -> vdq0/1
  Integrator/1 -> Gain2/1, Mux/1  "vd"
  Integrator3/1 -> Gain1/1, Mux/2  "vq"
  Add/1 -> Integrator/1
  Gain1/1 -> Add/2
  idq0/1 -> Demux/1
  1 / capacitance value d/1 -> Add/1
  Add1/1 -> Integrator3/1
  Gain2/1 -> Add1/1
  1 / capacitance value q/1 -> Add1/2
  1 / capacitance value 0/1 -> Integrator1/1
  Constant/1 -> Integrator/2
  Constant1/1 -> Integrator3/2
  Constant2/1 -> Integrator1/2
  Demux/1 -> 1 / capacitance value d/1  "id"
  Demux/2 -> 1 / capacitance value q/1  "iq"
  Demux/3 -> 1 / capacitance value 0/1  "i0"

== system ex7busLongLine_sim/shunt capacitor 6 ==
  note: dynamic model of balanced three-phase shunt capacitor unit, based on dq0 signals.
      | idq0 is the current flowing into the capacitor.
      | vdq0 is the capacitor voltage .
      | C is the capacitance (usually in F).
      | initial voltage - initial voltage on the capacitor (dq0 components).
  idq0 : Inport
  1 / capacitance value 0 : Gain  Gain=1/C6
  1 / capacitance value d : Gain  Gain=1/C6
  1 / capacitance value q : Gain  Gain=1/C6
  Add : Sum
  Add1 : Sum  Inputs=-+
  Constant : Constant  Value=(2^0.5)*Vbase
  Constant1 : Constant  Value=0
  Constant2 : Constant  Value=0
  Demux : Demux  Outputs=3
  Gain1 : Gain  Gain=ws
  Gain2 : Gain  Gain=ws
  Integrator : Integrator  InitialConditionSource=external  InitialCondition=bus1_vd
  Integrator1 : Integrator  InitialConditionSource=external  InitialCondition=bus1_vd
  Integrator3 : Integrator  InitialConditionSource=external  InitialCondition=bus1_vd
  Mux : Mux  Inputs=3
  vdq0 : Outport
  wires:
  Integrator1/1 -> Mux/3  "v0"
  Mux/1 -> vdq0/1
  Integrator/1 -> Gain2/1, Mux/1  "vd"
  Integrator3/1 -> Gain1/1, Mux/2  "vq"
  Add/1 -> Integrator/1
  Gain1/1 -> Add/2
  idq0/1 -> Demux/1
  1 / capacitance value d/1 -> Add/1
  Add1/1 -> Integrator3/1
  Gain2/1 -> Add1/1
  1 / capacitance value q/1 -> Add1/2
  1 / capacitance value 0/1 -> Integrator1/1
  Constant/1 -> Integrator/2
  Constant1/1 -> Integrator3/2
  Constant2/1 -> Integrator1/2
  Demux/1 -> 1 / capacitance value d/1  "id"
  Demux/2 -> 1 / capacitance value q/1  "iq"
  Demux/3 -> 1 / capacitance value 0/1  "i0"

== system ex7busLongLine_sim/shunt capacitor 2 ==
  note: dynamic model of balanced three-phase shunt capacitor unit, based on dq0 signals.
      | idq0 is the current flowing into the capacitor.
      | vdq0 is the capacitor voltage .
      | C is the capacitance (usually in F).
      | initial voltage - initial voltage on the capacitor (dq0 components).
  idq0 : Inport
  1 / capacitance value 0 : Gain  Gain=1/C2
  1 / capacitance value d : Gain  Gain=1/C2
  1 / capacitance value q : Gain  Gain=1/C2
  Add : Sum
  Add1 : Sum  Inputs=-+
  Constant : Constant  Value=(2^0.5)*Vbase
  Constant1 : Constant  Value=0
  Constant2 : Constant  Value=0
  Demux : Demux  Outputs=3
  Gain1 : Gain  Gain=ws
  Gain2 : Gain  Gain=ws
  Integrator : Integrator  InitialConditionSource=external  InitialCondition=bus1_vd
  Integrator1 : Integrator  InitialConditionSource=external  InitialCondition=bus1_vd
  Integrator3 : Integrator  InitialConditionSource=external  InitialCondition=bus1_vd
  Mux : Mux  Inputs=3
  vdq0 : Outport
  wires:
  Integrator1/1 -> Mux/3  "v0"
  Mux/1 -> vdq0/1
  Integrator/1 -> Gain2/1, Mux/1  "vd"
  Integrator3/1 -> Gain1/1, Mux/2  "vq"
  Add/1 -> Integrator/1
  Gain1/1 -> Add/2
  idq0/1 -> Demux/1
  1 / capacitance value d/1 -> Add/1
  Add1/1 -> Integrator3/1
  Gain2/1 -> Add1/1
  1 / capacitance value q/1 -> Add1/2
  1 / capacitance value 0/1 -> Integrator1/1
  Constant/1 -> Integrator/2
  Constant1/1 -> Integrator3/2
  Constant2/1 -> Integrator1/2
  Demux/1 -> 1 / capacitance value d/1  "id"
  Demux/2 -> 1 / capacitance value q/1  "iq"
  Demux/3 -> 1 / capacitance value 0/1  "i0"

== system ex7busLongLine_sim/shunt capacitor 3 ==
  note: dynamic model of balanced three-phase shunt capacitor unit, based on dq0 signals.
      | idq0 is the current flowing into the capacitor.
      | vdq0 is the capacitor voltage .
      | C is the capacitance (usually in F).
      | initial voltage - initial voltage on the capacitor (dq0 components).
  idq0 : Inport
  1 / capacitance value 0 : Gain  Gain=1/C3
  1 / capacitance value d : Gain  Gain=1/C3
  1 / capacitance value q : Gain  Gain=1/C3
  Add : Sum
  Add1 : Sum  Inputs=-+
  Constant : Constant  Value=(2^0.5)*Vbase
  Constant1 : Constant  Value=0
  Constant2 : Constant  Value=0
  Demux : Demux  Outputs=3
  Gain1 : Gain  Gain=ws
  Gain2 : Gain  Gain=ws
  Integrator : Integrator  InitialConditionSource=external  InitialCondition=bus1_vd
  Integrator1 : Integrator  InitialConditionSource=external  InitialCondition=bus1_vd
  Integrator3 : Integrator  InitialConditionSource=external  InitialCondition=bus1_vd
  Mux : Mux  Inputs=3
  vdq0 : Outport
  wires:
  Integrator1/1 -> Mux/3  "v0"
  Mux/1 -> vdq0/1
  Integrator/1 -> Gain2/1, Mux/1  "vd"
  Integrator3/1 -> Gain1/1, Mux/2  "vq"
  Add/1 -> Integrator/1
  Gain1/1 -> Add/2
  idq0/1 -> Demux/1
  1 / capacitance value d/1 -> Add/1
  Add1/1 -> Integrator3/1
  Gain2/1 -> Add1/1
  1 / capacitance value q/1 -> Add1/2
  1 / capacitance value 0/1 -> Integrator1/1
  Constant/1 -> Integrator/2
  Constant1/1 -> Integrator3/2
  Constant2/1 -> Integrator1/2
  Demux/1 -> 1 / capacitance value d/1  "id"
  Demux/2 -> 1 / capacitance value q/1  "iq"
  Demux/3 -> 1 / capacitance value 0/1  "i0"

== system ex7busLongLine_sim/shunt capacitor 4 ==
  note: dynamic model of balanced three-phase shunt capacitor unit, based on dq0 signals.
      | idq0 is the current flowing into the capacitor.
      | vdq0 is the capacitor voltage .
      | C is the capacitance (usually in F).
      | initial voltage - initial voltage on the capacitor (dq0 components).
  idq0 : Inport
  1 / capacitance value 0 : Gain  Gain=1/C4
  1 / capacitance value d : Gain  Gain=1/C4
  1 / capacitance value q : Gain  Gain=1/C4
  Add : Sum
  Add1 : Sum  Inputs=-+
  Constant : Constant  Value=(2^0.5)*Vbase
  Constant1 : Constant  Value=0
  Constant2 : Constant  Value=0
  Demux : Demux  Outputs=3
  Gain1 : Gain  Gain=ws
  Gain2 : Gain  Gain=ws
  Integrator : Integrator  InitialConditionSource=external  InitialCondition=bus1_vd
  Integrator1 : Integrator  InitialConditionSource=external  InitialCondition=bus1_vd
  Integrator3 : Integrator  InitialConditionSource=external  InitialCondition=bus1_vd
  Mux : Mux  Inputs=3
  vdq0 : Outport
  wires:
  Integrator1/1 -> Mux/3  "v0"
  Mux/1 -> vdq0/1
  Integrator/1 -> Gain2/1, Mux/1  "vd"
  Integrator3/1 -> Gain1/1, Mux/2  "vq"
  Add/1 -> Integrator/1
  Gain1/1 -> Add/2
  idq0/1 -> Demux/1
  1 / capacitance value d/1 -> Add/1
  Add1/1 -> Integrator3/1
  Gain2/1 -> Add1/1
  1 / capacitance value q/1 -> Add1/2
  1 / capacitance value 0/1 -> Integrator1/1
  Constant/1 -> Integrator/2
  Constant1/1 -> Integrator3/2
  Constant2/1 -> Integrator1/2
  Demux/1 -> 1 / capacitance value d/1  "id"
  Demux/2 -> 1 / capacitance value q/1  "iq"
  Demux/3 -> 1 / capacitance value 0/1  "i0"

== system ex7busLongLine_sim/shunt capacitor 7 ==
  note: dynamic model of balanced three-phase shunt capacitor unit, based on dq0 signals.
      | idq0 is the current flowing into the capacitor.
      | vdq0 is the capacitor voltage .
      | C is the capacitance (usually in F).
      | initial voltage - initial voltage on the capacitor (dq0 components).
  idq0 : Inport
  1 / capacitance value 0 : Gain  Gain=1/C7
  1 / capacitance value d : Gain  Gain=1/C7
  1 / capacitance value q : Gain  Gain=1/C7
  Add : Sum
  Add1 : Sum  Inputs=-+
  Constant : Constant  Value=(2^0.5)*Vbase
  Constant1 : Constant  Value=0
  Constant2 : Constant  Value=0
  Demux : Demux  Outputs=3
  Gain1 : Gain  Gain=ws
  Gain2 : Gain  Gain=ws
  Integrator : Integrator  InitialConditionSource=external  InitialCondition=bus1_vd
  Integrator1 : Integrator  InitialConditionSource=external  InitialCondition=bus1_vd
  Integrator3 : Integrator  InitialConditionSource=external  InitialCondition=bus1_vd
  Mux : Mux  Inputs=3
  vdq0 : Outport
  wires:
  Integrator1/1 -> Mux/3  "v0"
  Mux/1 -> vdq0/1
  Integrator/1 -> Gain2/1, Mux/1  "vd"
  Integrator3/1 -> Gain1/1, Mux/2  "vq"
  Add/1 -> Integrator/1
  Gain1/1 -> Add/2
  idq0/1 -> Demux/1
  1 / capacitance value d/1 -> Add/1
  Add1/1 -> Integrator3/1
  Gain2/1 -> Add1/1
  1 / capacitance value q/1 -> Add1/2
  1 / capacitance value 0/1 -> Integrator1/1
  Constant/1 -> Integrator/2
  Constant1/1 -> Integrator3/2
  Constant2/1 -> Integrator1/2
  Demux/1 -> 1 / capacitance value d/1  "id"
  Demux/2 -> 1 / capacitance value q/1  "iq"
  Demux/3 -> 1 / capacitance value 0/1  "i0"

== system ex7busLongLine_sim/switched resistive load 2 ==
  note: connected=0   -->   resistor disconnected, zero current
      | connected=1   -->   resistor connected
      |
      | current positive when flowing from the resistor into the grid
  vdq0 : Inport
  connected : Inport  Port=2
  1/R : Gain  Gain=-1/2.5e3
  Index Vector : MultiPortSwitch  DataPortOrder=Zero-based contiguous  Inputs=2  zeroidx=on
  cnst : Constant  Value=0
  idq0 : Outport
  wires:
  connected/1 -> Index Vector/1
  Index Vector/1 -> idq0/1
  vdq0/1 -> 1/R/1
  1/R/1 -> Index Vector/3
  cnst/1 -> Index Vector/2

== system ex7busLongLine_sim/switched resistive load 3 ==
  note: connected=0   -->   resistor disconnected, zero current
      | connected=1   -->   resistor connected
      |
      | current positive when flowing from the resistor into the grid
  vdq0 : Inport
  connected : Inport  Port=2
  1/R : Gain  Gain=-1/2.5e3
  Index Vector : MultiPortSwitch  DataPortOrder=Zero-based contiguous  Inputs=2  zeroidx=on
  cnst : Constant  Value=0
  idq0 : Outport
  wires:
  connected/1 -> Index Vector/1
  Index Vector/1 -> idq0/1
  vdq0/1 -> 1/R/1
  1/R/1 -> Index Vector/3
  cnst/1 -> Index Vector/2

== system ex7busLongLine_sim/switched resistive load 6 ==
  note: connected=0   -->   resistor disconnected, zero current
      | connected=1   -->   resistor connected
      |
      | current positive when flowing from the resistor into the grid
  vdq0 : Inport
  connected : Inport  Port=2
  1/R : Gain  Gain=-1/2.5e3
  Index Vector : MultiPortSwitch  DataPortOrder=Zero-based contiguous  Inputs=2  zeroidx=on
  cnst : Constant  Value=0
  idq0 : Outport
  wires:
  connected/1 -> Index Vector/1
  Index Vector/1 -> idq0/1
  vdq0/1 -> 1/R/1
  1/R/1 -> Index Vector/3
  cnst/1 -> Index Vector/2

== system ex7busLongLine_sim/switched resistive load 7 ==
  note: connected=0   -->   resistor disconnected, zero current
      | connected=1   -->   resistor connected
      |
      | current positive when flowing from the resistor into the grid
  vdq0 : Inport
  connected : Inport  Port=2
  1/R : Gain  Gain=-1/2.5e3
  Index Vector : MultiPortSwitch  DataPortOrder=Zero-based contiguous  Inputs=2  zeroidx=on
  cnst : Constant  Value=0
  idq0 : Outport
  wires:
  connected/1 -> Index Vector/1
  Index Vector/1 -> idq0/1
  vdq0/1 -> 1/R/1
  1/R/1 -> Index Vector/3
  cnst/1 -> Index Vector/2

== system ex7busLongLine_sim/transmission line 1-->2 ==
  note: sending
      | end
  note: receiving
      | end
  note: currents positive when flowing
      | into the line
  note: receiving
      | end
  note: sending
      | end
  vr : Inport
  vs : Inport  Port=2
  Demux : Demux  Outputs=2
  Mux : Mux  Inputs=2
  State-Space : StateSpace  A=full(At12)  B=full(Bt12)  C=full(Ct12)  D=full(Dt12)  X0=0
  ir : Outport
  is : Outport  Port=2
  wires:
  vs/1 -> Mux/1
  vr/1 -> Mux/2
  State-Space/1 -> Demux/1
  Demux/1 -> is/1
  Demux/2 -> ir/1
  Mux/1 -> State-Space/1

== system ex7busLongLine_sim/transmission line 1-->4 ==
  note: sending
      | end
  note: receiving
      | end
  note: currents positive when flowing
      | into the line
  note: receiving
      | end
  note: sending
      | end
  vr : Inport
  vs : Inport  Port=2
  Demux : Demux  Outputs=2
  Mux : Mux  Inputs=2
  State-Space : StateSpace  A=full(At14)  B=full(Bt14)  C=full(Ct14)  D=full(Dt14)  X0=0
  ir : Outport
  is : Outport  Port=2
  wires:
  vs/1 -> Mux/1
  vr/1 -> Mux/2
  State-Space/1 -> Demux/1
  Demux/1 -> is/1
  Demux/2 -> ir/1
  Mux/1 -> State-Space/1

== system ex7busLongLine_sim/transmission line 2-->3 ==
  note: sending
      | end
  note: receiving
      | end
  note: currents positive when flowing
      | into the line
  note: receiving
      | end
  note: sending
      | end
  vs : Inport
  vr : Inport  Port=2
  Demux : Demux  Outputs=2
  Mux : Mux  Inputs=2
  State-Space : StateSpace  A=full(At23)  B=full(Bt23)  C=full(Ct23)  D=full(Dt23)  X0=0
  is : Outport
  ir : Outport  Port=2
  wires:
  vs/1 -> Mux/1
  vr/1 -> Mux/2
  State-Space/1 -> Demux/1
  Demux/1 -> is/1
  Demux/2 -> ir/1
  Mux/1 -> State-Space/1

== system ex7busLongLine_sim/transmission line 2-->5 ==
  note: sending
      | end
  note: receiving
      | end
  note: currents positive when flowing
      | into the line
  note: receiving
      | end
  note: sending
      | end
  vr : Inport
  vs : Inport  Port=2
  Demux : Demux  Outputs=2
  Mux : Mux  Inputs=2
  State-Space : StateSpace  A=full(At25)  B=full(Bt25)  C=full(Ct25)  D=full(Dt25)  X0=0
  ir : Outport
  is : Outport  Port=2
  wires:
  vs/1 -> Mux/1
  vr/1 -> Mux/2
  State-Space/1 -> Demux/1
  Demux/1 -> is/1
  Demux/2 -> ir/1
  Mux/1 -> State-Space/1

== system ex7busLongLine_sim/transmission line 3-->4 ==
  note: sending
      | end
  note: receiving
      | end
  note: currents positive when flowing
      | into the line
  note: receiving
      | end
  note: sending
      | end
  vs : Inport
  vr : Inport  Port=2
  Demux : Demux  Outputs=2
  Mux : Mux  Inputs=2
  State-Space : StateSpace  A=full(At34)  B=full(Bt34)  C=full(Ct34)  D=full(Dt34)  X0=0
  is : Outport
  ir : Outport  Port=2
  wires:
  vs/1 -> Mux/1
  vr/1 -> Mux/2
  State-Space/1 -> Demux/1
  Demux/1 -> is/1
  Demux/2 -> ir/1
  Mux/1 -> State-Space/1

== system ex7busLongLine_sim/transmission line 4-->6 ==
  note: sending
      | end
  note: receiving
      | end
  note: currents positive when flowing
      | into the line
  note: receiving
      | end
  note: sending
      | end
  vr : Inport
  vs : Inport  Port=2
  Demux : Demux  Outputs=2
  Mux : Mux  Inputs=2
  State-Space : StateSpace  A=full(At46)  B=full(Bt46)  C=full(Ct46)  D=full(Dt46)  X0=0
  ir : Outport
  is : Outport  Port=2
  wires:
  vs/1 -> Mux/1
  vr/1 -> Mux/2
  State-Space/1 -> Demux/1
  Demux/1 -> is/1
  Demux/2 -> ir/1
  Mux/1 -> State-Space/1

== system ex7busLongLine_sim/transmission line 6-->7 ==
  note: sending
      | end
  note: receiving
      | end
  note: currents positive when flowing
      | into the line
  note: receiving
      | end
  note: sending
      | end
  vr : Inport
  vs : Inport  Port=2
  Demux : Demux  Outputs=2
  Mux : Mux  Inputs=2
  State-Space : StateSpace  A=full(At67)  B=full(Bt67)  C=full(Ct67)  D=full(Dt67)  X0=0
  ir : Outport
  is : Outport  Port=2
  wires:
  vs/1 -> Mux/1
  vr/1 -> Mux/2
  State-Space/1 -> Demux/1
  Demux/1 -> is/1
  Demux/2 -> ir/1
  Mux/1 -> State-Space/1
